simulink model "modulation_531"  (R2022b)
settings: Solver=VariableStepAuto  StartTime=0.0  StopTime=20  RelTol=1e-3
values from neighbouring files (symbols this model uses):
  A_c = 1    [main.m]    (also in test_model_validity.m)
  f_c = 10    [main.m]    (also in test_model_validity.m)
  f_m = rate    [main.m]    (also in test_model_validity.m)
  f_s = 20    [main.m]    (also in test_model_validity.m)
  k_f = 7.5    [main.m]    (also in test_model_validity.m)
settings Model: Creator=HaByeongchan  LastModifiedBy=HaByeongchan

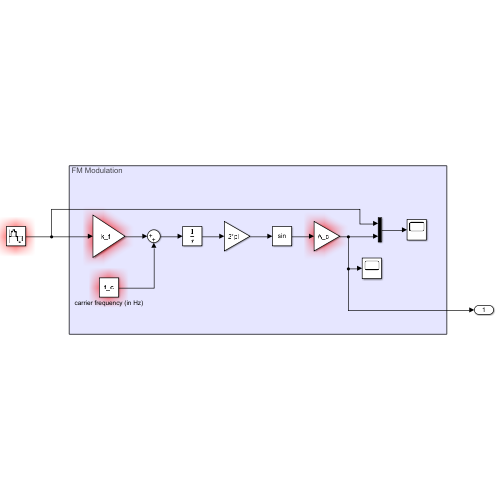
[thumbnail: Simulink's stored preview of the top-level diagram]
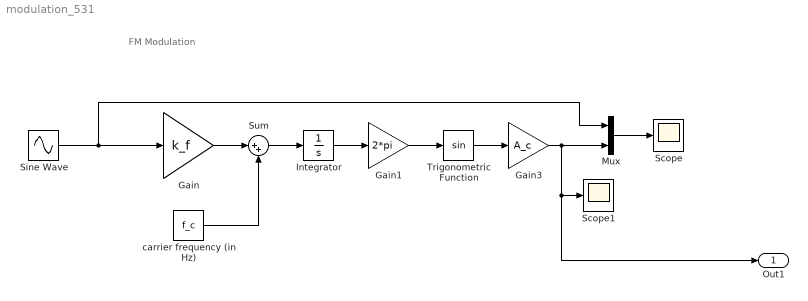
== system modulation_531 ==
  note: FM Modulation
  Gain : Gain  Gain=k_f
  Gain1 : Gain  Gain=2*pi
  Gain3 : Gain  Gain=A_c
  Integrator : Integrator
  Mux : Mux  Inputs=2
  Scope : Scope
  Scope1 : Scope
  Sine Wave : Sin  Frequency=f_m * 2 * pi  SampleTime=1/f_s
  Sum : Sum  Inputs=|++
  Trigonometric Function : Trigonometry
  carrier frequency (in Hz) : Constant  Value=f_c
  Out1 : Outport
  wires:
  Integrator/1 -> Gain1/1
  Mux/1 -> Scope/1
  Trigonometric Function/1 -> Gain3/1
  Gain1/1 -> Trigonometric Function/1
  carrier frequency (in Hz)/1 -> Sum/2
  Sum/1 -> Integrator/1
  Gain3/1 -> Out1/1, Scope1/1, Mux/2
  Sine Wave/1 -> Mux/1, Gain/1
  Gain/1 -> Sum/1
